simulink model "CarClosedLoop"  (Simulink 7.7)
settings: Solver=ode45  StartTime=0.0  StopTime=60.0  RelTol=1e-3
values from neighbouring files (symbols this model uses):
  den = ctr.den{1}    [car1.m]    (also in car2.m; car3.m; car4.m; pendulum.m)
  num = ctr.num{1}    [car1.m]    (also in car2.m; car3.m; car4.m; pendulum.m = K * ctr.num{1})
libraries: simulink x1
settings Model: Creator=mauricio  LastModifiedBy=mauricio

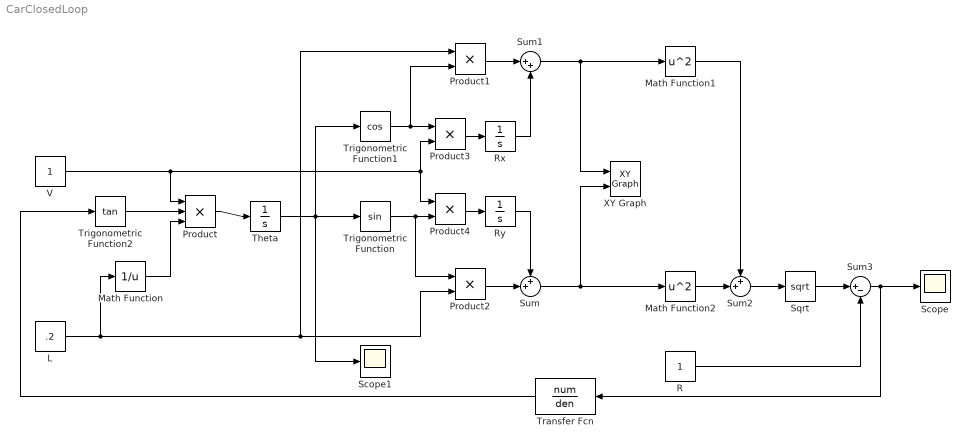
== system CarClosedLoop ==
  L : Constant  Value=.2
  Math Function : Math  Operator=reciprocal  SaturateOnIntegerOverflow=on
  Math Function1 : Math  Operator=square  SaturateOnIntegerOverflow=on
  Math Function2 : Math  Operator=square  SaturateOnIntegerOverflow=on
  Product : Product  Inputs=3  RndMeth=Zero
  Product{1..4} (4 alike) : Product  RndMeth=Zero
  R : Constant
  Rx : Integrator
  Ry : Integrator
  Scope : Scope
      settings: YMin=-0.8  YMax=0.7
  Scope1 : Scope
      settings: YMin=-10  YMax=150
  Sqrt : Sqrt  SaturateOnIntegerOverflow=on
  Sum : Sum  Inputs=++|
  Sum1 : Sum  Inputs=|++
  Sum2 : Sum  Inputs=++|
  Sum3 : Sum  Inputs=|+-
  Theta : Integrator
  Transfer Fcn : TransferFcn  Numerator=num  Denominator=den
  Trigonometric Function : Trigonometry
  Trigonometric Function1 : Trigonometry  Operator=cos
  Trigonometric Function2 : Trigonometry  Operator=tan
  V : Constant
  XY Graph : simulink/Sinks/XY Graph  SystemSampleTime=-1  xmin=-2  xmax=2  ymin=-2  ymax=2  st=-1
  wires:
  Trigonometric Function1/1 -> Product1/2, Product3/1
  Trigonometric Function/1 -> Product2/1, Product4/2
  Theta/1 -> Trigonometric Function/1, Trigonometric Function1/1, Scope1/1
  Product/1 -> Theta/1
  Rx/1 -> Sum1/2
  Ry/1 -> Sum/1
  L/1 -> Math Function/1, Product2/2, Product1/1
  Product1/1 -> Sum1/1
  Product2/1 -> Sum/2
  Sum1/1 -> XY Graph/1, Math Function1/1
  Sum/1 -> XY Graph/2, Math Function2/1
  Math Function2/1 -> Sum2/2
  Math Function1/1 -> Sum2/1
  Sum2/1 -> Sqrt/1
  Sqrt/1 -> Sum3/1
  R/1 -> Sum3/2
  Sum3/1 -> Scope/1, Transfer Fcn/1
  Product4/1 -> Ry/1
  Product3/1 -> Rx/1
  V/1 -> Product3/2, Product4/1, Product/1
  Trigonometric Function2/1 -> Product/2
  Math Function/1 -> Product/3
  Transfer Fcn/1 -> Trigonometric Function2/1
